simulink model "untitled"  (R2014a)
settings: Solver=VariableStepDiscrete  StartTime=0.0  StopTime=800  RelTol=1e-3
settings Model: Creator=ZJK  LastModifiedBy=ZJK

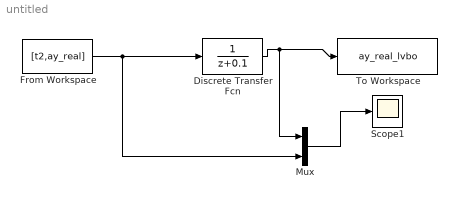
== system untitled ==
  Discrete Transfer Fcn : DiscreteTransferFcn  Denominator=[1 0.1]  SampleTime=0.01
  From Workspace : FromWorkspace  VariableName=[t2,ay_real]  SampleTime=0.01
  Mux : Mux  Inputs=2
  Scope1 : Scope
      settings: TickLabels=on
  To Workspace : ToWorkspace  VariableName=ay_real_lvbo  SaveFormat=Timeseries  SampleTime=-1
  wires:
  Discrete Transfer Fcn/1 -> Mux/1, To Workspace/1
  From Workspace/1 -> Mux/2, Discrete Transfer Fcn/1
  Mux/1 -> Scope1/1
